simulink model "TLS"  (R2020b)
settings: Solver=FixedStepAuto  StartTime=0.0  StopTime=Inf  RelTol=1e-3
PostLoadFcn:
  | if any(exist('dsrtsu_mdlpostloadfcn', 'file') ~= 0), dsrtsu_mdlpostloadfcn('Execute', bdroot); end
InitFcn:
  | , if any(exist('dsmpb_private', 'file') ~= 0), dsmpb_private('dsmpb_mdlclblib', 'Init', bdroot); end,
PreSaveFcn:
  | , if any(exist('dsmpb_private', 'file') ~= 0), dsmpb_private('dsmpb_mdlclblib', 'PreSave', bdroot); end,
CloseFcn:
  | , if any(exist('dsmpb_private', 'file') ~= 0), dsmpb_private('dsmpb_mdlclblib', 'Close', bdroot); end,
settings Model: DataDictionary=HWA_DDs.sldd  RTICANMMDATA=struct('GeneralSetupData',struct('modelroot',['E:\Feature\Lateral mode\ADAS_Store\ADAS_Store\Adas\VSM\LSSState\TargetLineSelect'],'generalsettings',struct('filesettings',struct('destfolder',struct('Name','RTICANMM_FILES','Check',1),'buildfolder',struct('Name','.','Check',1),'AbsDestfolder',struct('Name',['E:\Feature\Lateral mode\ADAS_Store\ADAS_Store\Adas\VSM\LSSState\TargetLineSelect\RTICANMM_FILES']),'AbsBuildfolder',struct('Name',['E:\Feature\Lateral mode\ADAS_Store\ADAS_Store\Adas\VSM\LSSState\TargetLineSelect']))),'options',struct('addpaths',1,'rmpaths',1,'addtrcexclusion',false,'cannavigator',struct('checkmonitoring',0),'show_usrtrc',0,'use_usrtrc',0),'advanced',struct('options',ones(1,100)),'MPSetup',{{}},'RTI',struct('Type','DSRT','Ver','4.2','Date','02-Nov-2019'),'modelname','TLS','block','TLS'))  DSRTSU_INTERNAL_RTIFPGA=150  Creator=GW00164453  LastModifiedBy=GW00164453
settings OptimizationCC: BlockReduction=off  ConditionallyExecuteInputs=off  OptimizeBlockIOStorage=off  BufferReuse=off
settings DebuggingCC: TasksWithSamePriorityMsg=none
settings HardwareCC: ProdBitPerPointer=32  ProdBitPerSizeT=32  ProdBitPerPtrDiffT=32  ProdLargestAtomicInteger=Integer  ProdWordSize=32  ProdHWDeviceType=Custom Processor->Custom
settings ModelReferenceCC: UpdateModelReferenceTargets=IfOutOfDate  EnableParallelModelReferenceBuilds=on  ModelReferenceNumInstancesAllowed=Single
settings SFSimCC: MATLABDynamicMemAlloc=off
settings RTWCC: Description=dSPACE Run-Time Target (for VEOS on Windows and ConfigurationDesk)  SystemTargetFile=dsrt.tlc  GenCodeOnly=on  MakeCommand=make_dsrt  TemplateMakefile=dsrt_default_tmf  RTWVerbose=off
settings CodeAppCC: MaxIdLength=128
settings STFCustomTargetCC: TargetLangStandard=C99 (ISO)  ParMdlRefBuildCompliant=on  ConcurrentExecutionCompliant=off  CPPClassGenCompliant=off  GRTInterface=off  SystemTargetFile=dsrt.tlc
settings GRTTargetCC: CompOptLevelCompliant=off  ConcurrentExecutionCompliant=off  CombineOutputUpdateFcns=off  MatFileLogging=off  CPPClassGenCompliant=off  UseToolchainInfoCompliant=off

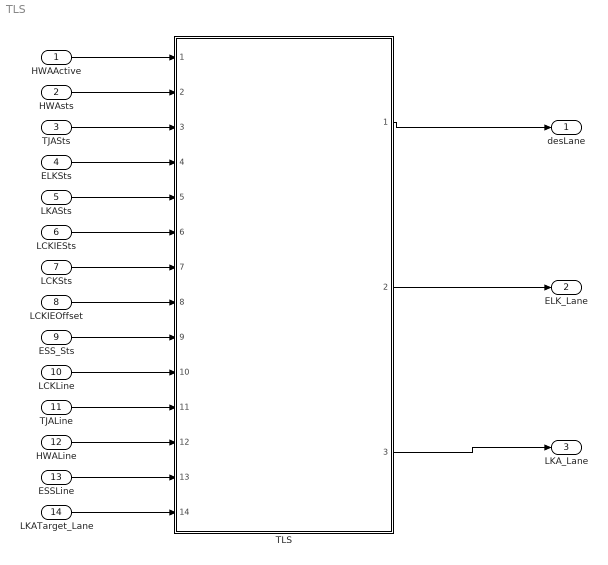
== system TLS ==
  HWAActive : Inport
  HWAsts : Inport  Port=2  OutDataTypeStr=Enum: HWA_STATE
  TJASts : Inport  Port=3  OutDataTypeStr=Enum: TJA_STATE
  "ELKSts " : Inport  Port=4  OutDataTypeStr=Enum: ELKSTATE
  LKASts : Inport  Port=5  OutDataTypeStr=Enum: STATE
  LCKIESts : Inport  Port=6  OutDataTypeStr=Enum: STATE
  LCKSts : Inport  Port=7  OutDataTypeStr=Enum: LCK_STATE
  LCKIEOffset : Inport  Port=8
  "ESS_Sts " : Inport  Port=9
  LCKLine : Inport  Port=10  OutDataTypeStr=Bus: LSM_LCK_BUS
  TJALine : Inport  Port=11  OutDataTypeStr=Bus: LSM_TJA_ICA_BUS
  HWALine : Inport  Port=12  OutDataTypeStr=Bus: LSM_HWA_BUS
  ESSLine : Inport  Port=13  OutDataTypeStr=Bus: LSM_ESS_BUS
  "LKATarget_Lane " : Inport  Port=14  OutDataTypeStr=Bus: LaneARe_SP
  TLS : Subsystem  ReferencedSubsystem=SubSystem_VSM_TLS
  desLane : Outport  OutDataTypeStr=Bus: TLS_DesLane
  ELK_Lane : Outport  Port=2  OutDataTypeStr=Bus: TLS_ELKLane
  LKA_Lane : Outport  Port=3  OutDataTypeStr=Bus: TLS_LKALane
  wires:
  HWAActive/1 -> TLS/1
  HWAsts/1 -> TLS/2
  TJASts/1 -> TLS/3
  "ELKSts "/1 -> TLS/4
  LKASts/1 -> TLS/5
  LCKIESts/1 -> TLS/6
  LCKSts/1 -> TLS/7
  LCKIEOffset/1 -> TLS/8
  "ESS_Sts "/1 -> TLS/9
  LCKLine/1 -> TLS/10
  TJALine/1 -> TLS/11
  HWALine/1 -> TLS/12
  ESSLine/1 -> TLS/13
  "LKATarget_Lane "/1 -> TLS/14
  TLS/2 -> ELK_Lane/1
  TLS/1 -> desLane/1
  TLS/3 -> LKA_Lane/1
